simulink model "Excavator_Mevea_BucketDriveline"  (R2026a)
settings: Solver=ode23t  StopTime=29.5  FixedStep=1e-5  MaxStep=Ts  AbsTol=1e-3
PostLoadFcn:
  | set_param(bdroot,'IgnoredZcDiagnostic','none');
  | Excavator_Test_Scenario_Select('loadedBucketDigCycle');
  | Excavator_Mevea_params
StartFcn:
  | tic
StopFcn:
  | elapsedSimTime = toc;
  | disp(['Elapsed Sim Time = ' num2str(elapsedSimTime)]);
model workspace: external: MAT-File ExcavatorAssemblyDataStruct.mat (data not in the file)
undefined symbols (not defined in the file or in its folder): AToBRegOrificeVector, AToTOrificeVector, BiPOrificeVector, BoomC, boomHEArea, boomREArea, boomUpMaxQ, boomValve, BToTOrificeVector, BucketC, bucketCloseMaxQ, bucketOpenMaxQ, BucketR, bucketValve, DiscIntNeverNeededParam, fluids, gravity, K, Lambda, LeftBoomR, maxPumpDisp, minPumpDisp, nominalEngineSpeed, P28Assembly, PToAOrificeVector, PToBOrificeVector, pumpCmdNegRateLimit, pumpCmdPosRateLimit, RightBoomR, StickC, stickInMaxQ, stickOutMaxQ, StickR, stickValve, SwingC, swingDisplacement, swingHighSpeedThreshold, swingMaxQ, SwingR, swingSpeedQGain, swingValve, tau, valveCmdNegRateLimit, valveCmdPosRateLimit, X, x0, Y, Z
libraries: fl_lib x113, SimscapeFluids_lib x78, nesl_utility x61, sm_lib x55, simulink_extras x11, Excavator_Parts_Lib x6, sm_wheel_loader_lib x6, simulink x5, sdl_lib x4, SignalEditorBlockLib x1
(part 8 of 8)

== system Excavator_Mevea_BucketDriveline/Excavator/Machine/Mevea/Interface CrawlerL/Port 1 Interface/Interface/Discrete ==
  across2 : Inport
  across1 : Inport  Port=2
  -1 : Gain  Gain=-1  SaturateOnIntegerOverflow=on  OutDataTypeStr=Inherit: Same as input  ParamDataTypeStr=Inherit: Same as input
  First-order lag : DiscreteTransferFcn  Numerator=h1  Denominator=[tau h1-tau]  SampleTime=h1
  Integrator : DiscreteIntegrator  InitialCondition=x0  SampleTime=h1  ICPrevOutput=DiscIntNeverNeededParam  ICPrevScaledInput=DiscIntNeverNeededParam
  K : Gain  Gain=K  SaturateOnIntegerOverflow=on  OutDataTypeStr=Inherit: Same as input  ParamDataTypeStr=Inherit: Same as input
  Lambda : Gain  Gain=Lambda  SaturateOnIntegerOverflow=on  OutDataTypeStr=Inherit: Same as input  ParamDataTypeStr=Inherit: Same as input
  Prediction : Subsystem  Commented=through  mask(Prediction (slow->fast)){h2=h2, h1=h1}
      mask prompts: h2 "physmod:simscape:couplers:SimscapeNetworkCouplersLib:PortUDiscreteSampleTimes_MP"; h1 "physmod:simscape:couplers:SimscapeNetworkCouplersLib:PortYDiscreteSampleTimes_MP"
      mask help: physmod:simscape:couplers:SimscapeNetworkCouplersLib:Predictionslowfast_MD
      mask DialogControl h2 Prompt: Port u discrete sample time (s)
      mask DialogControl h1 Prompt: Port y discrete sample time (s)
  Smoothing : Subsystem  Commented=through  mask(Smoothing (fast->slow)){nSmooth=nSmooth, h1=h1, smoothing0=-through0}
      mask prompts: nSmooth "physmod:simscape:couplers:SimscapeNetworkCouplersLib:NumberOfSamplesOverWhichToSmooth_MP"; h1 "physmod:simscape:couplers:SimscapeNetworkCouplersLib:PortUDiscreteSampleTimes_MP"; smoothing0 "physmod:simscape:couplers:SimscapeNetworkCouplersLib:InitialOutput_MP"
      mask help: physmod:simscape:couplers:SimscapeNetworkCouplersLib:Smoothingfastslow_MD
      mask DialogControl nSmooth Prompt: Number of samples over which to smooth
      mask DialogControl h1 Prompt: Port u discrete sample time (s)
      mask DialogControl smoothing0 Prompt: Initial output
  Sum : Sum  Inputs=+-  InputSameDT=on  SaturateOnIntegerOverflow=on  OutDataTypeStr=Inherit: Same as first input
  Sum1 : Sum  Inputs=|++
  through2 : Outport
  through1 : Outport  Port=2
  wires:
  -1/1 -> Smoothing/1(u)
  Smoothing/1(y) -> through2/1
  Prediction/1(y) -> Sum/2
  Lambda/1 -> Sum1/2
  Sum1/1 -> -1/1, through1/1
  across2/1 -> Prediction/1(u)
  Sum/1 -> First-order lag/1, Integrator/1
  across1/1 -> Sum/1
  K/1 -> Sum1/1
  Integrator/1 -> K/1
  First-order lag/1 -> Lambda/1

== system Excavator_Mevea_BucketDriveline/Excavator/Machine/Mevea/Interface CrawlerR/Port 1 Interface/Interface/Continuous ==
  across2 : Inport
  across1 : Inport  Port=2
  -1 : Gain  Gain=-1  SaturateOnIntegerOverflow=on  OutDataTypeStr=Inherit: Same as input  ParamDataTypeStr=Inherit: Same as input
  Integrator : Integrator  InitialCondition=x0
  K : Gain  Gain=K  SaturateOnIntegerOverflow=on  OutDataTypeStr=Inherit: Same as input  ParamDataTypeStr=Inherit: Same as input
  Lambda : Gain  Gain=Lambda  SaturateOnIntegerOverflow=on  OutDataTypeStr=Inherit: Same as input  ParamDataTypeStr=Inherit: Same as input
  Low-pass filter : TransferFcn  Numerator=1  Denominator=[tau 1]
  Prediction : Subsystem  Commented=through  mask(Prediction (discrete->continuous)){h2=h2}
      mask prompts: h2 "physmod:simscape:couplers:SimscapeNetworkCouplersLib:PortUDiscreteSampleTimes_MP"
      mask help: physmod:simscape:couplers:SimscapeNetworkCouplersLib:Predictiondiscretecontinuous_MD
      mask DialogControl h2 Prompt: Port u discrete sample time (s)
  Smoothing : Subsystem  Commented=through  mask(Smoothing (continuous->discrete)){tsSmoothing=tsSmoothing, smoothing0=-through0}
      mask prompts: tsSmoothing "physmod:simscape:couplers:SimscapeNetworkCouplersLib:SmoothingTimeConstants_MP"; smoothing0 "physmod:simscape:couplers:SimscapeNetworkCouplersLib:InitialOutput_MP"
      mask help: physmod:simscape:couplers:SimscapeNetworkCouplersLib:Smoothingcontinuousdiscrete_MD
      mask DialogControl tsSmoothing Prompt: Smoothing time constant (s)
      mask DialogControl smoothing0 Prompt: Initial output
  Sum : Sum  Inputs=+-  InputSameDT=on  SaturateOnIntegerOverflow=on  OutDataTypeStr=Inherit: Same as first input
  Sum2 : Sum  Inputs=|++
  through2 : Outport
  through1 : Outport  Port=2
  wires:
  -1/1 -> Smoothing/1(u)
  Smoothing/1(y) -> through2/1
  Prediction/1(y) -> Sum/2
  Lambda/1 -> Sum2/2
  across1/1 -> Sum/1
  Sum/1 -> Low-pass filter/1, Integrator/1
  Integrator/1 -> K/1
  Low-pass filter/1 -> Lambda/1
  across2/1 -> Prediction/1(u)
  Sum2/1 -> -1/1, through1/1
  K/1 -> Sum2/1

== system Excavator_Mevea_BucketDriveline/Excavator/Machine/Mevea/Interface CrawlerR/Port 1 Interface/Interface/Discrete ==
  across2 : Inport
  across1 : Inport  Port=2
  -1 : Gain  Gain=-1  SaturateOnIntegerOverflow=on  OutDataTypeStr=Inherit: Same as input  ParamDataTypeStr=Inherit: Same as input
  First-order lag : DiscreteTransferFcn  Numerator=h1  Denominator=[tau h1-tau]  SampleTime=h1
  Integrator : DiscreteIntegrator  InitialCondition=x0  SampleTime=h1  ICPrevOutput=DiscIntNeverNeededParam  ICPrevScaledInput=DiscIntNeverNeededParam
  K : Gain  Gain=K  SaturateOnIntegerOverflow=on  OutDataTypeStr=Inherit: Same as input  ParamDataTypeStr=Inherit: Same as input
  Lambda : Gain  Gain=Lambda  SaturateOnIntegerOverflow=on  OutDataTypeStr=Inherit: Same as input  ParamDataTypeStr=Inherit: Same as input
  Prediction : Subsystem  Commented=through  mask(Prediction (slow->fast)){h2=h2, h1=h1}
      mask prompts: h2 "physmod:simscape:couplers:SimscapeNetworkCouplersLib:PortUDiscreteSampleTimes_MP"; h1 "physmod:simscape:couplers:SimscapeNetworkCouplersLib:PortYDiscreteSampleTimes_MP"
      mask help: physmod:simscape:couplers:SimscapeNetworkCouplersLib:Predictionslowfast_MD
      mask DialogControl h2 Prompt: Port u discrete sample time (s)
      mask DialogControl h1 Prompt: Port y discrete sample time (s)
  Smoothing : Subsystem  Commented=through  mask(Smoothing (fast->slow)){nSmooth=nSmooth, h1=h1, smoothing0=-through0}
      mask prompts: nSmooth "physmod:simscape:couplers:SimscapeNetworkCouplersLib:NumberOfSamplesOverWhichToSmooth_MP"; h1 "physmod:simscape:couplers:SimscapeNetworkCouplersLib:PortUDiscreteSampleTimes_MP"; smoothing0 "physmod:simscape:couplers:SimscapeNetworkCouplersLib:InitialOutput_MP"
      mask help: physmod:simscape:couplers:SimscapeNetworkCouplersLib:Smoothingfastslow_MD
      mask DialogControl nSmooth Prompt: Number of samples over which to smooth
      mask DialogControl h1 Prompt: Port u discrete sample time (s)
      mask DialogControl smoothing0 Prompt: Initial output
  Sum : Sum  Inputs=+-  InputSameDT=on  SaturateOnIntegerOverflow=on  OutDataTypeStr=Inherit: Same as first input
  Sum1 : Sum  Inputs=|++
  through2 : Outport
  through1 : Outport  Port=2
  wires:
  -1/1 -> Smoothing/1(u)
  Smoothing/1(y) -> through2/1
  Prediction/1(y) -> Sum/2
  Lambda/1 -> Sum1/2
  Sum1/1 -> -1/1, through1/1
  across2/1 -> Prediction/1(u)
  Sum/1 -> First-order lag/1, Integrator/1
  across1/1 -> Sum/1
  K/1 -> Sum1/1
  Integrator/1 -> K/1
  First-order lag/1 -> Lambda/1

== system Excavator_Mevea_BucketDriveline/Excavator/Machine/Mevea/Interface CrawlerL/Port 1 Interface/Interface/Continuous/Prediction ==
  u : Inport
  1/h2 : Gain  Gain=1/h2
  Constant : Constant  SampleTime=h2
  Constant1 : Constant  Value=0  SampleTime=h2
  Constant2 : Constant  SampleTime=h2
  "Delay " : Delay  DelayLength=1  SampleTime=h2
  Delay 1 : Delay  DelayLength=1  SampleTime=h2
  Ignore the first output : Switch  Criteria=u2 > Threshold  SaturateOnIntegerOverflow=off  InputSameDT=off
  Integrator : Integrator  ExternalReset=either  LimitOutput=on  UpperSaturationLimit=1  LowerSaturationLimit=0
  Product : Product
  Pulse Generator : DiscretePulseGenerator  SampleTime=h2
  Sum : Sum  Inputs=|++
  Sum4 : Sum  Inputs=+-|
  Zero-Order Hold : ZeroOrderHold  SampleTime=h2
  y : Outport
  wires:
  Constant2/1 -> Delay 1/1
  Delay 1/1 -> Ignore the first output/2
  Constant1/1 -> Ignore the first output/3
  Sum4/1 -> Ignore the first output/1
  Ignore the first output/1 -> 1/h2/1
  Pulse Generator/1 -> Integrator/2
  Constant/1 -> Integrator/1
  Integrator/1 -> Product/2  "Resetting ramp"
  Sum/1 -> y/1
  1/h2/1 -> Product/1  "Derivative"
  "Delay "/1 -> Sum4/2
  u/1 -> Zero-Order Hold/1, Sum/1
  Zero-Order Hold/1 -> "Delay "/1, Sum4/1
  Product/1 -> Sum/2  "Inter-sample prediction"

== system Excavator_Mevea_BucketDriveline/Excavator/Machine/Mevea/Interface CrawlerL/Port 1 Interface/Interface/Continuous/Smoothing ==
  u : Inport
  Gain : Gain  Gain=1/tsSmoothing
  Integrator : Integrator  InitialCondition=smoothing0
  Sum : Sum  Inputs=|+-
  y : Outport
  wires:
  Sum/1 -> Gain/1
  Gain/1 -> Integrator/1
  Integrator/1 -> y/1, Sum/2
  u/1 -> Sum/1

== system Excavator_Mevea_BucketDriveline/Excavator/Machine/Mevea/Interface CrawlerL/Port 1 Interface/Interface/Discrete/Prediction ==
  u : Inport
  Abs : Abs  SaturateOnIntegerOverflow=off
  Constant : Constant  Value=0  SampleTime=h1
  Constant2 : Constant  Value=h1  SampleTime=h1
  "Delay " : Delay  DelayLength=1  SampleTime=h1
  Product : Product
  Resettable Delay : Delay  DelayLength=1  InitialConditionSource=Input port  ExternalReset=Rising  SampleTime=h1
      settings: InputPortMap=u0,r5,p4
  Sum : Sum  Inputs=|++
  Sum1 : Sum  Inputs=|++
  Sum2 : Sum  Inputs=+
  Sum4 : Sum  Inputs=+-|
  Update derivative estimate : Subsystem  TreatAsAtomicUnit=on
  y : Outport
  wires:
  Constant/1 -> Resettable Delay/3
  Constant2/1 -> Sum1/1
  Resettable Delay/1 -> Sum1/2, Product/2
  Sum4/1 -> Abs/1
  u/1 -> Sum4/1, Sum/1, "Delay "/1, Update derivative estimate/1(u)
  Update derivative estimate/1(Out1) -> Product/1
  Product/1 -> Sum/2
  "Delay "/1 -> Sum4/2
  Sum/1 -> y/1
  Sum1/1 -> Resettable Delay/1
  Sum2/1 -> Update derivative estimate/Trigger, Resettable Delay/2  "Trigger when input changes"
  Abs/1 -> Sum2/1

== system Excavator_Mevea_BucketDriveline/Excavator/Machine/Mevea/Interface CrawlerL/Port 1 Interface/Interface/Discrete/Smoothing ==
  u : Inport
  Gain : Gain  Gain=1/nSmooth
  Sum of Elements : Sum  Inputs=+
  Tapped Delay : simulink/Discrete/Tapped Delay  vinit=smoothing0  samptime=h1  NumDelays=nSmooth  DelayOrder=Oldest  includeCurrent=off
  y : Outport
  wires:
  u/1 -> Tapped Delay/1
  Tapped Delay/1 -> Sum of Elements/1
  Sum of Elements/1 -> Gain/1
  Gain/1 -> y/1

== system Excavator_Mevea_BucketDriveline/Excavator/Machine/Mevea/Interface CrawlerR/Port 1 Interface/Interface/Continuous/Prediction ==
  u : Inport
  1/h2 : Gain  Gain=1/h2
  Constant : Constant  SampleTime=h2
  Constant1 : Constant  Value=0  SampleTime=h2
  Constant2 : Constant  SampleTime=h2
  "Delay " : Delay  DelayLength=1  SampleTime=h2
  Delay 1 : Delay  DelayLength=1  SampleTime=h2
  Ignore the first output : Switch  Criteria=u2 > Threshold  SaturateOnIntegerOverflow=off  InputSameDT=off
  Integrator : Integrator  ExternalReset=either  LimitOutput=on  UpperSaturationLimit=1  LowerSaturationLimit=0
  Product : Product
  Pulse Generator : DiscretePulseGenerator  SampleTime=h2
  Sum : Sum  Inputs=|++
  Sum4 : Sum  Inputs=+-|
  Zero-Order Hold : ZeroOrderHold  SampleTime=h2
  y : Outport
  wires:
  Constant2/1 -> Delay 1/1
  Delay 1/1 -> Ignore the first output/2
  Constant1/1 -> Ignore the first output/3
  Sum4/1 -> Ignore the first output/1
  Ignore the first output/1 -> 1/h2/1
  Pulse Generator/1 -> Integrator/2
  Constant/1 -> Integrator/1
  Integrator/1 -> Product/2  "Resetting ramp"
  Sum/1 -> y/1
  1/h2/1 -> Product/1  "Derivative"
  "Delay "/1 -> Sum4/2
  u/1 -> Zero-Order Hold/1, Sum/1
  Zero-Order Hold/1 -> "Delay "/1, Sum4/1
  Product/1 -> Sum/2  "Inter-sample prediction"

== system Excavator_Mevea_BucketDriveline/Excavator/Machine/Mevea/Interface CrawlerR/Port 1 Interface/Interface/Continuous/Smoothing ==
  u : Inport
  Gain : Gain  Gain=1/tsSmoothing
  Integrator : Integrator  InitialCondition=smoothing0
  Sum : Sum  Inputs=|+-
  y : Outport
  wires:
  Sum/1 -> Gain/1
  Gain/1 -> Integrator/1
  Integrator/1 -> y/1, Sum/2
  u/1 -> Sum/1

== system Excavator_Mevea_BucketDriveline/Excavator/Machine/Mevea/Interface CrawlerR/Port 1 Interface/Interface/Discrete/Prediction ==
  u : Inport
  Abs : Abs  SaturateOnIntegerOverflow=off
  Constant : Constant  Value=0  SampleTime=h1
  Constant2 : Constant  Value=h1  SampleTime=h1
  "Delay " : Delay  DelayLength=1  SampleTime=h1
  Product : Product
  Resettable Delay : Delay  DelayLength=1  InitialConditionSource=Input port  ExternalReset=Rising  SampleTime=h1
      settings: InputPortMap=u0,r5,p4
  Sum : Sum  Inputs=|++
  Sum1 : Sum  Inputs=|++
  Sum2 : Sum  Inputs=+
  Sum4 : Sum  Inputs=+-|
  Update derivative estimate : Subsystem  TreatAsAtomicUnit=on
  y : Outport
  wires:
  Constant/1 -> Resettable Delay/3
  Constant2/1 -> Sum1/1
  Resettable Delay/1 -> Sum1/2, Product/2
  Sum4/1 -> Abs/1
  u/1 -> Sum4/1, Sum/1, "Delay "/1, Update derivative estimate/1(u)
  Update derivative estimate/1(Out1) -> Product/1
  Product/1 -> Sum/2
  "Delay "/1 -> Sum4/2
  Sum/1 -> y/1
  Sum1/1 -> Resettable Delay/1
  Sum2/1 -> Update derivative estimate/Trigger, Resettable Delay/2  "Trigger when input changes"
  Abs/1 -> Sum2/1

== system Excavator_Mevea_BucketDriveline/Excavator/Machine/Mevea/Interface CrawlerR/Port 1 Interface/Interface/Discrete/Smoothing ==
  u : Inport
  Gain : Gain  Gain=1/nSmooth
  Sum of Elements : Sum  Inputs=+
  Tapped Delay : simulink/Discrete/Tapped Delay  vinit=smoothing0  samptime=h1  NumDelays=nSmooth  DelayOrder=Oldest  includeCurrent=off
  y : Outport
  wires:
  u/1 -> Tapped Delay/1
  Tapped Delay/1 -> Sum of Elements/1
  Sum of Elements/1 -> Gain/1
  Gain/1 -> y/1

== system Excavator_Mevea_BucketDriveline/Excavator/Machine/Mevea/Interface CrawlerL/Port 1 Interface/Interface/Discrete/Prediction/Update derivative estimate ==
  u : Inport
  Trigger : TriggerPort  VariantControl=(inherit)
  1/h2 : Gain  Gain=1/h2
  Constant : Constant  Value=0  SampleTime=-1
  Constant1 : Constant  SampleTime=-1
  Sum : Sum  Inputs=|-+
  Switch : Switch  Criteria=u2 > Threshold  SaturateOnIntegerOverflow=off  InputSameDT=off
  Unit Delay : UnitDelay  SampleTime=-1
  Wait one sample : UnitDelay  SampleTime=-1
  Out1 : Outport
  wires:
  Constant1/1 -> Wait one sample/1
  Wait one sample/1 -> Switch/2
  Constant/1 -> Switch/3
  Sum/1 -> Switch/1
  Switch/1 -> 1/h2/1
  1/h2/1 -> Out1/1
  u/1 -> Sum/2, Unit Delay/1
  Unit Delay/1 -> Sum/1

== system Excavator_Mevea_BucketDriveline/Excavator/Machine/Mevea/Interface CrawlerR/Port 1 Interface/Interface/Discrete/Prediction/Update derivative estimate ==
  u : Inport
  Trigger : TriggerPort  VariantControl=(inherit)
  1/h2 : Gain  Gain=1/h2
  Constant : Constant  Value=0  SampleTime=-1
  Constant1 : Constant  SampleTime=-1
  Sum : Sum  Inputs=|-+
  Switch : Switch  Criteria=u2 > Threshold  SaturateOnIntegerOverflow=off  InputSameDT=off
  Unit Delay : UnitDelay  SampleTime=-1
  Wait one sample : UnitDelay  SampleTime=-1
  Out1 : Outport
  wires:
  Constant1/1 -> Wait one sample/1
  Wait one sample/1 -> Switch/2
  Constant/1 -> Switch/3
  Sum/1 -> Switch/1
  Switch/1 -> 1/h2/1
  1/h2/1 -> Out1/1
  u/1 -> Sum/2, Unit Delay/1
  Unit Delay/1 -> Sum/1

== matlab function Excavator_Mevea_BucketDriveline/Controller/Function Commander/HydraulicCommander ==
  data: swingCmd input; boomCmd input; stickCmd input; bucketCmd input; swingQDmd output; stickHEPr input; stickREPr input; swingSpeed input; boomQDmd output; stickQDmd output; bucketQDmd output; leftPumpDispCmd output; rightPumpDispCmd output; swingMaxQ parameter; boomUpMaxQ parameter; stickOutMaxQ parameter; stickInMaxQ parameter; bucketCloseMaxQ parameter; bucketOpenMaxQ parameter; swingSpoolPos output; boomSpoolPos output; stickSpoolPos output; bucketSpoolPos output; shaftSpeed input; nominalShaftSpeed parameter; minPumpDisp parameter; maxPumpDisp parameter; swingSpeedQGain parameter; swingHighSpeedThreshold parameter
function [swingQDmd, boomQDmd, stickQDmd, bucketQDmd, leftPumpDispCmd, ...
    rightPumpDispCmd, swingSpoolPos, boomSpoolPos, stickSpoolPos, ...
    bucketSpoolPos] = HydraulicCommander( ...
    swingCmd, boomCmd, stickCmd, bucketCmd, stickHEPr, stickREPr, ...
    swingSpeed, swingMaxQ, boomUpMaxQ, stickOutMaxQ, stickInMaxQ, ...
    bucketCloseMaxQ, bucketOpenMaxQ, shaftSpeed, nominalShaftSpeed, ...
    minPumpDisp, maxPumpDisp, swingSpeedQGain, swingHighSpeedThreshold)
%% Initialization
% Flow Rate Demands
swingQDmd = 0; % [lpm]
boomQDmd = 0; % [lpm]
stickQDmd = 0; % [lpm]
bucketQDmd = 0; % [lpm]

% Spool Positions
swingSpoolPos = 0; % [mm]
boomSpoolPos = 0; % [mm]
stickSpoolPos = 0; % [mm]
bucketSpoolPos = 0; % [mm]

% Max Spool Positions
maxPosSpoolPos = 5; % [mm]
maxNegSpoolPos = -5; % [mm]

%% Swing Flow Rate Demand & Spool Position
% Flow Rate
if swingCmd ~= 0
    % Operator command flow rate
    swingOpCmdFlowRate = abs(swingCmd) * swingMaxQ; % [lpm]
  
    % If the swing speed is high or the swing command is opposing the 
    % current speed, use the flow rate directly proportional to the 
    % operator command
    if abs(swingSpeed) > swingHighSpeedThreshold || sign(swingCmd) == sign(swingSpeed)   
        swingQDmd = swingOpCmdFlowRate; % [lpm]
    else
        % Limit the swing flow rate demand based on the current swing speed
        % This limits the flow loss through the swing pressure relief valve
        % during acceleration
        swingSpeedLimitedFlowRate = abs(swingSpeed) * swingSpeedQGain; % [lpm]
        
        % Only use the limited value if it is less than the operator
        % command value
        if swingSpeedLimitedFlowRate < swingOpCmdFlowRate
            swingQDmd = swingSpeedLimitedFlowRate; % [lpm]
        else
            swingQDmd = swingOpCmdFlowRate; % [lpm]
        end
    end 
end

% Spool Position
% Swing Right
if swingCmd > 0
    swingSpoolPos = maxPosSpoolPos; % [mm]
% Swing Left
elseif swingCmd < 0
    swingSpoolPos = maxNegSpoolPos; % [mm]
end

%% Boom Flow Rate Demand & Spool Position
% Boom Up Command Logic - Active Flow
if boomCmd < 0
    boomQDmd = abs(boomCmd) * boomUpMaxQ; % [lpm]
    boomSpoolPos = maxNegSpoolPos; % [mm]
% Boom Down Command Logic - Regenerative Flow
elseif boomCmd > 0
    % For boom down, the valve spool position is varied based on the
    % operator command and there is no pump flow required due to the
    % regenerative flow valve allowing flow from the head end to the rod
    % end during the move. The spool position must be controlled in this 
    % case so that the speed of the boom is proportional to the command. 
    % For boom up, the speed is controlled by limiting the pump flow - but 
    % for boom down, because there is no pump flow, the valve must be used.
    boomSpoolPosFactor = interp1([0 0.10 0.20 0.30 0.40 0.50 0.60 0.70 0.80 0.90 1], ...
                                 [0 0.30 0.45 0.55 0.60 0.70 0.75 0.80 0.85 0.90 1], ...
                                  boomCmd); % [mm]
    boomSpoolPos = maxPosSpoolPos * boomSpoolPosFactor; % [mm]
end

%% Stick Flow Rate Demand & Spool Position
% Stick Out Command Logic - Active Flow
if stickCmd > 0
    stickQDmd = abs(stickCmd) * stickOutMaxQ; % [lpm]
    stickSpoolPos = maxPosSpoolPos; % [mm]
% Stick In Command Logic - Active & Regenerative Flow
elseif stickCmd < 0
    deltaPr = stickREPr - stickHEPr; % [bar]
    if deltaPr > 120
        % When the pressure difference is high, limit the pump flow rate
        % and valve opening to take advantage of the regenerative flow from
        % the rod end. If the valve is opened all the way with a high
        % difference in pressure, the stick velocity will be very high and
        % uncontrolled.  
        stickQDmdFactor = 0.15;
        stickSpoolPosFactor = interp1([0 1], [0 0.55], abs(stickCmd));
    elseif deltaPr > 15
        % When the pressure difference is moderate, start increasing the
        % valve area and pump flow to maintain the velocity.
        stickQDmdFactor = interp1([15 120], [1 0.15], abs(deltaPr));
        stickSpoolPosFactor = interp1([0 1], [0 0.75], abs(stickCmd));
    else
        % When the pressure difference is low, or the head end pressure is
        % higher than the rod end, open the valve completely and allow full
        % pump flow.
        stickQDmdFactor = 1;
        stickSpoolPosFactor = 1;
    end
    % Multiply the maximum flow rate and valve position commands by the
    % factors calculated above to obtain the desired values.
    stickQDmd = abs(stickCmd) * stickInMaxQ * stickQDmdFactor; % [lpm]
    stickSpoolPos = maxNegSpoolPos * stickSpoolPosFactor; % [mm]
end

%% Bucket Flow Rate Demand & Spool Position
% Bucket Open Command Logic - Active Flow
if bucketCmd > 0
    bucketQDmd = abs(bucketCmd) * bucketOpenMaxQ; % [lpm]
    bucketSpoolPos = maxPosSpoolPos; % [mm]
% Bucket Close Command Logic - Active Flow
elseif bucketCmd < 0
    bucketQDmd = abs(bucketCmd) * bucketCloseMaxQ; % [lpm]
    bucketSpoolPos = maxNegSpoolPos; % [mm]
end

%% Pump Distribution
% Max pump flow rate
maxRatedPumpQ = (nominalShaftSpeed * maxPumpDisp)/1000; % [lpm]

% Left Pump: Boom, Stick, Swing
leftPumpQDmd = boomQDmd/2 + stickQDmd/2 + swingQDmd; % [lpm]
% Saturate flow rate demand
if leftPumpQDmd > maxRatedPumpQ
    leftPumpQDmd = maxRatedPumpQ; % [lpm]
end

% Right Pump: Boom, Stick, Bucket
rightPumpQDmd = boomQDmd/2 + stickQDmd/2 + bucketQDmd; % [lpm]
% Saturate flow rate demand
if rightPumpQDmd > maxRatedPumpQ
    rightPumpQDmd = maxRatedPumpQ; % [lpm]
end

%% Left Pump Command
% Convert Flow Rate to Displacement
leftPumpDispCmd = 1000 * (leftPumpQDmd/shaftSpeed); % [cc/rev]
% Saturate displacement command
if leftPumpDispCmd < minPumpDisp
    leftPumpDispCmd = minPumpDisp; % [cc/rev]
elseif leftPumpDispCmd > maxPumpDisp
    leftPumpDispCmd = maxPumpDisp; % [cc/rev]
end

%% Right Pump Command
% Convert Flow Rate to Displacement
rightPumpDispCmd = 1000 * (rightPumpQDmd/shaftSpeed); % [cc/rev]
% Saturate displacement command
if rightPumpDispCmd < minPumpDisp
    rightPumpDispCmd = minPumpDisp; % [cc/rev]
elseif rightPumpDispCmd > maxPumpDisp
    rightPumpDispCmd = maxPumpDisp; % [cc/rev]
end
